simulink model "simulinkParkGarage"  (R2024a)
settings: Solver=VariableStepAuto  StartTime=0.0  StopTime=14.0333  RelTol=1e-3
values from neighbouring files (symbols this model uses):
  posX = [sampleTimes',position(:,1)]    [main.m]
  posY = [sampleTimes',position(:,2)]    [main.m]
  posYaw = [sampleTimes',yaw]    [main.m]
libraries: visionsinks x2, sim3dcameralib x1, sim3dlib x1, sim3dautolib x1
settings Model: Creator=Administrator  LastModifiedBy=6000022946

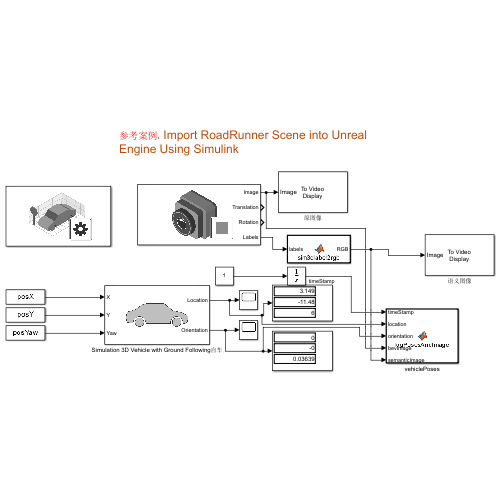
[thumbnail: Simulink's stored preview of the top-level diagram]
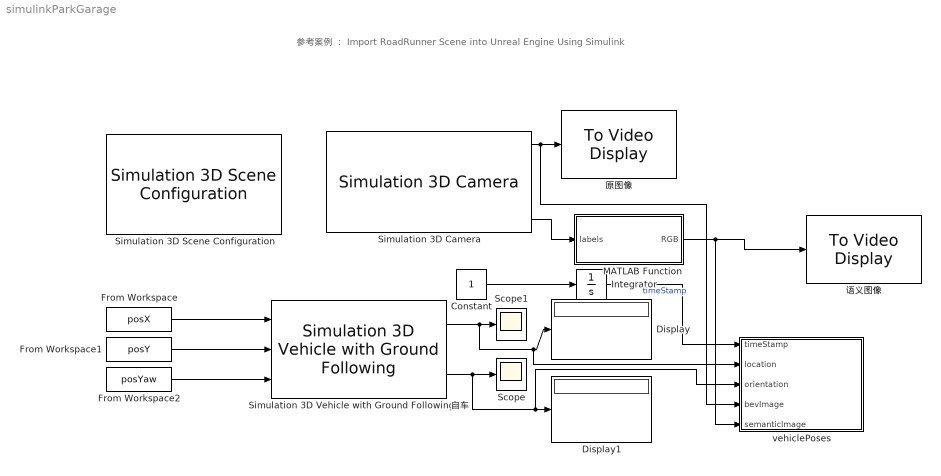
== system simulinkParkGarage ==
  note: 参考案例 ： Import RoadRunner Scene into Unreal Engine Using Simulink
  Constant : Constant
  Display : Display
  Display1 : Display
  From Workspace : FromWorkspace  VariableName=posX
  From Workspace1 : FromWorkspace  VariableName=posY
  From Workspace2 : FromWorkspace  VariableName=posYaw
  Integrator : Integrator
  MATLAB Function : MATLAB Function  TreatAsAtomicUnit=on
  Scope : Scope
  Scope1 : Scope
  Simulation 3D Camera : sim3dcameralib/Simulation 3D Camera  Priority=1  sensorTag=Sim3dSensor1  sensorId=1  sensorName=Sim3dSensor1  vehTagList={'Scene Origin';'SimulinkVehicle11'}  vehTag=SimulinkVehicle11  mountLoc=Origin  offsetFlag=on  tmountOffset=[0, 0, 2.4]  extTmount=off  rmountOffset=[0, 90, 0]  extRmount=off  FocalLength=[170, 170]  OpticalCenter=[540, 360]  ImageSize=[720, 1080]  RadialDistortion=[0, 0]  TangentialDistortion=[0, 0]  SensorSkew=0  DepthOutportEnabled=off  SemanticOutportEnabled=on  TransformOutportEnabled=on  SampleTime=-1  mountPoint=[0 0 2.4]  mountOrientation=[0 -90 0]  aMode=3  ID=1
      settings: LibrarySourceBlock=drivingsim3d/Simulation 3D Camera
  Simulation 3D Scene Configuration : sim3dlib/Simulation 3D Scene Configuration  Priority=0  ProjectFormat=RoadRunner  SceneDesc=Straight road  ProjectName=C:\Program Files\MATLAB\R2024a\toolbox\shared\sim3d_projects\automotive_project_windows\UE\WindowsNoEditor\VehicleSimulation.exe  ScenePath=/Game/Maps/HwStrght  RoadRunnerProjectPath=D:\roadrunner_works\New RoadRunner Project\Exports\ParkingGarage.fbx  EnableOpenDRIVE=off  vehTagList={'Custom';'Scene Origin';'SimulinkVehicle11'}  vehTag=SimulinkVehicle11  FreeCameraInitialTranslation=[50, 0, 200]  FreeCameraDefaultInitialTranslation=[-6, 0, 2]  FreeCameraInitialRotation=[0, -90, 0]  FreeCameraDefaultInitialRotation=[0, -15, 0]  OpVisEn=off  Ts=1/60  EnableWindow=on  EnableRemoteAccess=off  EnableWeather=on  SunAzimuth=90  SunAltitude=40.0  EnableGeospatialSun=off  Latitude=0  Longitude=0  Date=2023-01-01  Time=10:30:00  SunDaylightSaving=off  wind=4.0  clouds=89.0  EnableVolumetricClouds=on  CloudCoverage=0  CloudAltitude=6  fog=0.0  rain=0.0  RaindropsEffect=off  SnowDensity=0  EnableGeospatial=off  UseTrueOrigin=off  OriginHeight=200  OriginLatitude=40.744652  OriginLongitude=-73.988864  MapStyle=Aerial  AdditionalAssetIDs=[]  UseAdvancedSunSky=off  SolarTime=11  TimeZone=-5  Day=21  Month=9  Year=2022  UseDaylightSavingTime=on  DSTStartDay=10  DSTStartMonth=3  DSTEndDay=3  DSTEndMonth=11  DSTSwitchHour=2  sensorTag=MainCamera1  sensorId=1  sensorName=MainCamera1  mountLoc=Origin  offsetFlag=off  tmountOffset=[0, 0, 0]  rmountOffset=[0, 0, 0]  HorizontalResolution=1280  VerticalResolution=720  HorizontalFOV=60  mountPoint=[0 0 0]  mountOrientation=[0 0 0]  aMode=3  ID=1  GeoTrigger=Inactive
      settings: LibrarySourceBlock=drivingsim3d/Simulation 3D Scene Configuration
  Simulation 3D Vehicle with Ground Following自车 : sim3dautolib/Simulation 3D Vehicle with Ground Following  Priority=-1  PassVehMesh=Sedan  MeshPath=/MathWorksAutomotiveContent/Vehicles/Muscle/Meshes/SK_MuscleCar.SK_MuscleCar  TrackWidth=1.9  WheelBase=3  WheelRadius=0.35  VehColor=Red  InitialPos=[posX(1,2),posY(1,2),6]  InitialRot=[0, 0, posYaw(1,2)]  ActorName=SimulinkVehicle11  SampleTime=-1  ActorType=SimulinkVehicle  ID=11  aMode=3  ActorTag=SimulinkVehicle11  CoordinateScheme=ISO  VehLightsControl=off  HeadlightColor=[ 1, 1, 1 ]  HighBeamIntensity=100000  LowBeamIntensity=60000  HighBeamConeAngle=70  LowBeamConeAngle=70  LeftHeadlightOrientation=[ 0, 0 ]  RightHeadlightOrientation=[ 0, 0 ]  BrakelightIntensity=500  ReverselightIntensity=500  SignallightIntensity=500  SignallightPeriod=1  SignalPulseWidth=50  TransformOutportEnabled=on
      settings: LibrarySourceBlock=drivingsim3d/Simulation 3D Vehicle with Ground Following
  vehiclePoses : MATLAB Function  TreatAsAtomicUnit=on
  原图像 : visionsinks/To Video Display  windowSizeMode=Normal  openAtMdlStart=on  fullScreen=off  videoWindowX=64  videoWindowY=87  saveWindowSize=off  videoWindowWidth=1280  videoWindowHeight=720  inputColorFormat=RGB  inputType=Obsolete  imagePorts=One multidimensional signal  OutputDevice=On-screen video monitor  dataOrg=Column-major  isWindowOpen=off
  语义图像 : visionsinks/To Video Display  windowSizeMode=Normal  openAtMdlStart=on  fullScreen=off  videoWindowX=242  videoWindowY=274  saveWindowSize=off  videoWindowWidth=1280  videoWindowHeight=720  inputColorFormat=RGB  inputType=Obsolete  imagePorts=One multidimensional signal  OutputDevice=On-screen video monitor  dataOrg=Column-major  isWindowOpen=off
  wires:
  Simulation 3D Camera/1 -> vehiclePoses/4(bevImage), 原图像/1
  From Workspace/1 -> Simulation 3D Vehicle with Ground Following自车/1
  Simulation 3D Camera/4 -> MATLAB Function/1(labels)
  MATLAB Function/1(RGB) -> vehiclePoses/5(semanticImage), 语义图像/1
  Simulation 3D Vehicle with Ground Following自车/1 -> vehiclePoses/2(location), Display/1, Scope1/1
  Simulation 3D Vehicle with Ground Following自车/2 -> vehiclePoses/3(orientation), Display1/1, Scope/1
  From Workspace1/1 -> Simulation 3D Vehicle with Ground Following自车/2
  From Workspace2/1 -> Simulation 3D Vehicle with Ground Following自车/3
  Integrator/1 -> vehiclePoses/1(timeStamp)  "timeStamp"
  Constant/1 -> Integrator/1

== matlab function simulinkParkGarage/MATLAB Function ==
  data: labels input; RGB output
function RGB = sim3dlabel2rgb(labels)
% Convert semantic segmentation map captured during 3D simulation to RGB
% color image.

% Declare label2rgb function.
coder.extrinsic('label2rgb');

% Preallocate memory for RGB matrix.
RGB = coder.nullcopy(zeros(size(labels,1),size(labels,2),3,class(labels)));

% Define colormap using 3D simulation label IDs.
cmap = sim3dColormap;

% Convert labels to RGB color image.
RGB = label2rgb(labels, cmap,'c');

== matlab function simulinkParkGarage/vehiclePoses ==
  data: timeStamp input; location input; orientation input; bevImage input; semanticImage input
function logPosesAndImage(timeStamp,location, orientation,bevImage,semanticImage)
% matlab function block使用，用于曾总Simulation 3D Camera 模块实时仿真输出存储，2024.1.26
coder.extrinsic("logSensorSubFcn");
logSensorSubFcn(timeStamp,location, orientation,bevImage,semanticImage);
end
